simulink model "oscillator"  (Simulink 9.2)
settings: Solver=VariableStepAuto  StartTime=0.0  StopTime=20  RelTol=1e-3
values from neighbouring files (symbols this model uses):
  C = 0.25    [constants.m]    (also in problem1.m)
  L = 1.6    [constants.m]    (also in problem1.m)
  R1 = 4    [constants.m]    (also in problem1.m)
  R2 = 2    [constants.m]    (also in estimate_price.m = 1 - (SSE/SST); problem1.m)
  R3 = 3    [constants.m]    (also in problem1.m)
settings Model: Creator=Henkka  LastModifiedBy=Henkka
settings DataIOCC: LimitDataPoints=off  SaveFormat=Dataset  SignalLoggingSaveFormat=Dataset
settings OptimizationCC: LifeSpan=auto
settings DebuggingCC: UnderspecifiedInitializationDetection=Simplified  MergeDetectMultiDrivingBlocksExec=error  FcnCallInpInsideContextMsg=error  StateNameClashWarn=none  SFUnexpectedBacktrackingDiag=error  SFNoUnconditionalDefaultTransitionDiag=error  SFExecutionAtInitializationDiag=warning
settings HardwareCC: ProdBitPerPointer=64  ProdBitPerSizeT=64  ProdBitPerPtrDiffT=64  ProdLargestAtomicFloat=Float  ProdIntDivRoundTo=Zero  ProdEndianess=LittleEndian  ProdWordSize=64  ProdHWDeviceType=Intel->x86-64 (Windows64)
settings ModelReferenceCC: PropagateSignalLabelsOutOfModel=on
settings SFSimCC: SimUseLocalCustomCode=on
settings RTWCC: RTWUseLocalCustomCode=on
settings CodeAppCC: StateflowObjectComments=off
settings GRTTargetCC: TargetLangStandard=C99 (ISO)  GeneratePreprocessorConditionals=Use local settings  CombineOutputUpdateFcns=on  GRTInterface=off
settings ConfigComp: CovMetricSettings=dwe  CovHtmlReporting=off  CovSaveCumulativeToWorkspaceVar=off  CovSaveSingleToWorkspaceVar=off  CovExternalEMLEnable=on

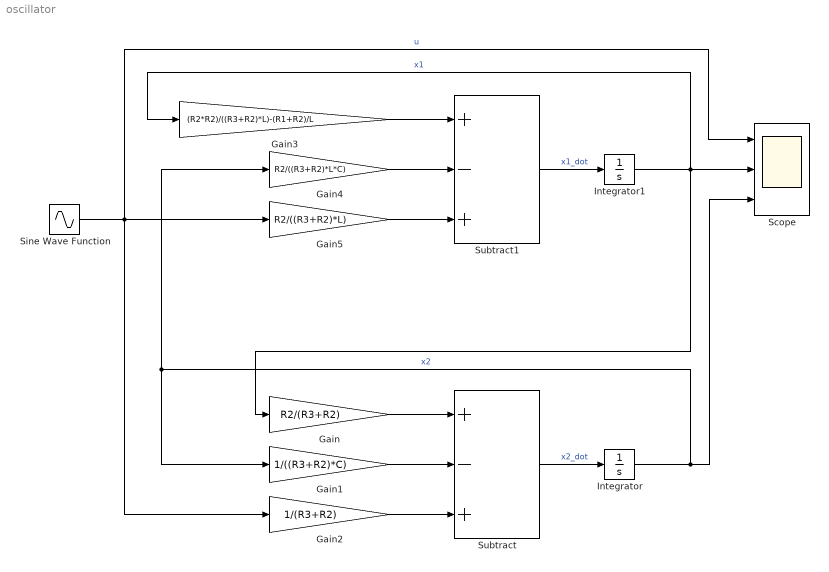
== system oscillator ==
  Gain : Gain  Gain=R2/(R3+R2)
  Gain1 : Gain  Gain=1/((R3+R2)*C)
  Gain2 : Gain  Gain=1/(R3+R2)
  Gain3 : Gain  Gain=(R2*R2)/((R3+R2)*L)-(R1+R2)/L
  Gain4 : Gain  Gain=R2/((R3+R2)*L*C)
  Gain5 : Gain  Gain=R2/((R3+R2)*L)
  Integrator : Integrator  InitialCondition=2  ContinuousStateAttributes='q'
  Integrator1 : Integrator  InitialCondition=15  ContinuousStateAttributes='I_1'
  Scope : Scope  NumInputPorts=3
  Sine Wave Function : Sin  SampleTime=0
  Subtract : Sum  Inputs=+-+
  Subtract1 : Sum  Inputs=+-+
  wires:
  Sine Wave Function/1 -> Gain2/1, Scope/1, Gain5/1  "u"
  Gain2/1 -> Subtract/3
  Gain1/1 -> Subtract/2
  Gain/1 -> Subtract/1
  Subtract/1 -> Integrator/1  "x2_dot"
  Integrator/1 -> Gain1/1, Gain4/1, Scope/3  "x2"
  Gain3/1 -> Subtract1/1
  Gain5/1 -> Subtract1/3
  Gain4/1 -> Subtract1/2
  Subtract1/1 -> Integrator1/1  "x1_dot"
  Integrator1/1 -> Gain/1, Gain3/1, Scope/2  "x1"
